simulink model "algebraicLoop_example"  (R2016b)
settings: Solver=FixedStepDiscrete  StartTime=0.0  StopTime=10.0  RelTol=1e-3
settings Model: Creator=hbourbou  LastModifiedBy=hbourbou

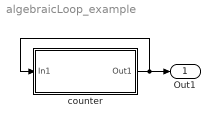
== system algebraicLoop_example ==
  counter : Subsystem
  Out1 : Outport
  wires:
  counter/1(Out1) -> Out1/1, counter/1(In1)

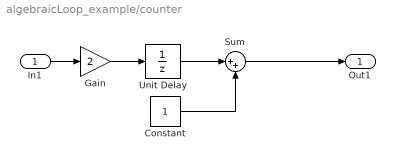
== system algebraicLoop_example/counter ==
  In1 : Inport
  Constant : Constant
  Gain : Gain  Gain=2
  Sum : Sum  Inputs=|++
  Unit Delay : UnitDelay  SampleTime=-1  HasFrameUpgradeWarning=on
  Out1 : Outport
  wires:
  Sum/1 -> Out1/1
  In1/1 -> Gain/1
  Unit Delay/1 -> Sum/1
  Constant/1 -> Sum/2
  Gain/1 -> Unit Delay/1
